simulink model "MotorSim_MechanicalParameterEstimation"  (R2019b)
settings: Solver=VariableStepAuto  StartTime=0.0  StopTime=2*ramp_time  MaxStep=5e-5  RelTol=1e-3
PreLoadFcn:
  | modelDir = fileparts(get_param(bdroot, 'FileName'));
  | addpath(fullfile(modelDir,'../Parameters'));
  | addpath(fullfile(modelDir,'subsystems'));
  | 
  | Parameters_Model
  | Parameters_Simulation
  | Parameters_Test_Ramp
InitFcn:
  | Parameters_Model
  | Parameters_Simulation
  | Parameters_Test_Ramp
undefined symbols (not defined in the file): ramp_duty_end, ramp_duty_start, ramp_steps, ramp_time, Vbat
libraries: simulink x2
settings Model: Creator=Thomas  LastModifiedBy=thomas.jespersen
settings DataIOCC: ReturnWorkspaceOutputs=off
settings DebuggingCC: ArithmeticOperatorsInVariantConditions=warning
settings SFSimCC: SimUseLocalCustomCode=off  CustomCodeUndefinedFunction=UseInterfaceOnly
settings RTWCC: RTWUseLocalCustomCode=off

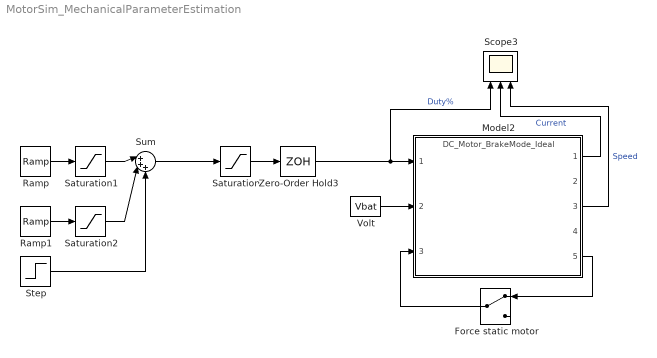
== system MotorSim_MechanicalParameterEstimation ==
  Force static motor : ManualSwitch
  Model2 : ModelReference  ModelNameDialog=DC_Motor_BrakeMode_Ideal  SimulationMode=Normal  ModelReferenceVersion=1.26
  Ramp : simulink/Sources/Ramp  slope=(ramp_duty_end-ramp_duty_start)/((ramp_time/ramp_steps)*(ramp_steps-1))  start=0  InitialOutput=ramp_duty_start
  Ramp1 : simulink/Sources/Ramp  slope=(ramp_duty_end-ramp_duty_start)/((ramp_time/ramp_steps)*(ramp_steps-1))  start=ramp_time  InitialOutput=0
  Saturation : Saturate  UpperLimit=1  LowerLimit=-1
  Saturation1 : Saturate  UpperLimit=max(ramp_duty_start, ramp_duty_end)  LowerLimit=min(ramp_duty_start, ramp_duty_end)
  Saturation2 : Saturate  UpperLimit=max(ramp_duty_start, ramp_duty_end)  LowerLimit=min(ramp_duty_start, ramp_duty_end)
  Scope3 : Scope  NumInputPorts=3
  Step : Step  Time=ramp_time  After=-2*ramp_duty_end  SampleTime=0
  Sum : Sum  Inputs=|+++
  Volt : Constant  Value=Vbat
  Zero-Order Hold3 : ZeroOrderHold  SampleTime=ramp_time/(ramp_steps+1)
  wires:
  Volt/1 -> Model2/2
  Force static motor/1 -> Model2/3
  Model2/5 -> Force static motor/1
  Saturation/1 -> Zero-Order Hold3/1
  Zero-Order Hold3/1 -> Scope3/1, Model2/1  "Duty%"
  Model2/1 -> Scope3/2  "Current"
  Model2/3 -> Scope3/3  "Speed"
  Ramp1/1 -> Saturation2/1
  Sum/1 -> Saturation/1
  Saturation1/1 -> Sum/1
  Ramp/1 -> Saturation1/1
  Saturation2/1 -> Sum/2
  Step/1 -> Sum/3
